simulink model "DevLib_PwrStgState"  (R2016b)
settings: configuration reference "CodeGenConfigSet" (kept outside this file)
values from neighbouring files (symbols this model uses):
  DebLib_facPwrStgHighHysHi_C = Calibration.Parameter    [init_DevLib_PwrStgState.m]
  DebLib_facPwrStgHighHysLo_C = Calibration.Parameter    [init_DevLib_PwrStgState.m]
  DebLib_facPwrStgLowHysHi_C = Calibration.Parameter    [init_DevLib_PwrStgState.m]
  DebLib_facPwrStgLowHysLo_C = Calibration.Parameter    [init_DevLib_PwrStgState.m]
  DebLib_uBattThdBattHiHysHi_C = Calibration.Parameter    [init_DevLib_PwrStgState.m]
  DebLib_uBattThdBattHiHysLo_C = Calibration.Parameter    [init_DevLib_PwrStgState.m]
  DebLib_uBattThdBattLoHysHi_C = Calibration.Parameter    [init_DevLib_PwrStgState.m]
  DebLib_uBattThdBattLoHysLo_C = Calibration.Parameter    [init_DevLib_PwrStgState.m]
  DebLib_uPwrStgBattHiHysHi_C = Calibration.Parameter    [init_DevLib_PwrStgState.m]
  DebLib_uPwrStgBattHiHysLo_C = Calibration.Parameter    [init_DevLib_PwrStgState.m]
  DebLib_uPwrStgBattLoHysHi_C = Calibration.Parameter    [init_DevLib_PwrStgState.m]
  DebLib_uPwrStgBattLoHysLo_C = Calibration.Parameter    [init_DevLib_PwrStgState.m]
undefined symbols (not defined in the file or in its folder): SubSysExeState_conv
libraries: simulink x13, CXLib x6
settings Model: Creator=lenovo  LastModifiedBy=lenovo
settings ConfigSetRef: SourceLocation=Base Workspace

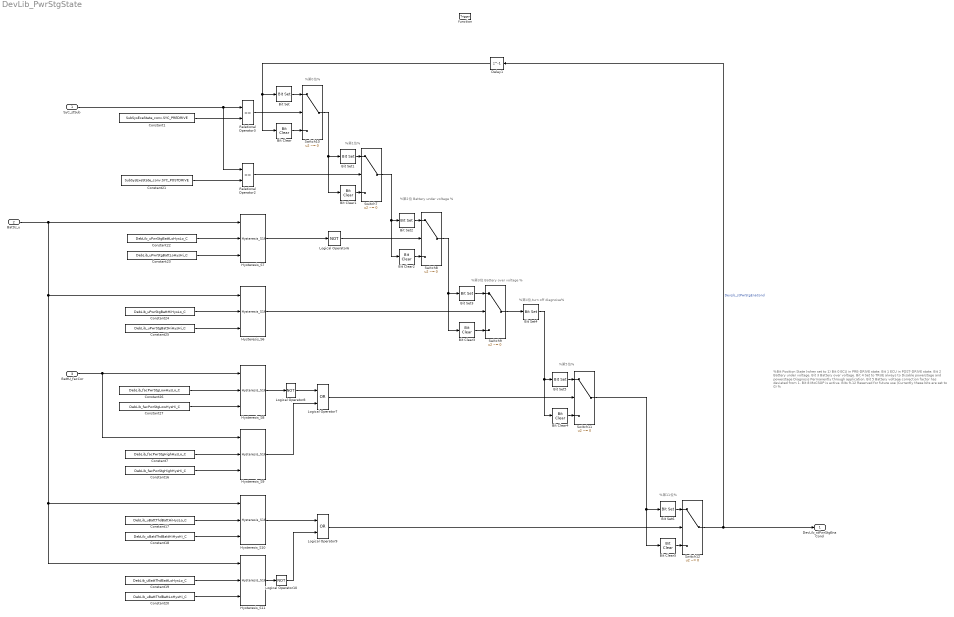
== system DevLib_PwrStgState ==
  note: %第11位%
  note: %第5位%
  note: %第4位,turn off diagnoise%
  note: %第3位 Battery over voltage %
  note: %第2位 Battery under voltage %
  note: %第1位%
  note: %第0位%
  note: %Bit Position State (when set to 1)
      | Bit 0 ECU in PRE-DRIVE state.
      | Bit 1 ECU in POST-DRIVE state.
      | Bit 2 Battery under voltage.
      | Bit 3 Battery over voltage.
      | Bit 4 Set to TRUE always to Disable powerstage and powerstage Diagnosis Permanently through application.
      | Bit 5 Battery voltage correction factor has deviated from 1.
      | Bit 8 MoCSOP is active.
      | Bits 9-12 Reserved for future use (Currently these bits are set to 0) %
  SyC_stSub : Inport  Description=Current system/ECU sub-state  OutDataTypeStr=Enum: SubSysExeState_conv
  BattU_u : Inport  Tag=mv  Description=Battery voltage  Port=2  OutMin=0  OutMax=50000  OutDataTypeStr=Battery_mv
  BattU_facCor : Inport  Description=Battery correction factor  Port=3  OutMin=-32  OutMax=31.9  OutDataTypeStr=Factor
  function : TriggerPort  TriggerType=function-call  VariantControl=Variant
  Bit Clear : simulink/Logic and Bit Operations/Bit Clear  iBit=0
  Bit Clear1 : simulink/Logic and Bit Operations/Bit Clear  iBit=1
  Bit Clear2 : simulink/Logic and Bit Operations/Bit Clear  iBit=2
  Bit Clear3 : simulink/Logic and Bit Operations/Bit Clear  iBit=3
  Bit Clear4 : simulink/Logic and Bit Operations/Bit Clear  iBit=5
  Bit Clear5 : simulink/Logic and Bit Operations/Bit Clear  iBit=11
  Bit Set : simulink/Logic and Bit Operations/Bit Set  iBit=0
  Bit Set1 : simulink/Logic and Bit Operations/Bit Set  iBit=1
  Bit Set2 : simulink/Logic and Bit Operations/Bit Set  iBit=2
  Bit Set3 : simulink/Logic and Bit Operations/Bit Set  iBit=3
  Bit Set4 : simulink/Logic and Bit Operations/Bit Set  iBit=4
  Bit Set5 : simulink/Logic and Bit Operations/Bit Set  iBit=5
  Bit Set6 : simulink/Logic and Bit Operations/Bit Set  iBit=11
  Constant1 : Constant  Value=SubSysExeState_conv.SYC_PREDRIVE  SampleTime=-1
  Constant16 : Constant  Value=DebLib_facPwrStgHighHysHi_C  SampleTime=-1
  Constant17 : Constant  Value=DebLib_uBattThdBattHiHysLo_C  VectorParams1D=off  SampleTime=-1
  Constant18 : Constant  Value=DebLib_uBattThdBattHiHysHi_C  SampleTime=-1
  Constant19 : Constant  Value=DebLib_uBattThdBattLoHysLo_C  VectorParams1D=off  SampleTime=-1
  Constant20 : Constant  Value=DebLib_uBattThdBattLoHysHi_C  SampleTime=-1
  Constant21 : Constant  Value=SubSysExeState_conv.SYC_POSTDRIVE  SampleTime=-1
  Constant22 : Constant  Value=DebLib_uPwrStgBattLoHysLo_C  SampleTime=-1
  Constant23 : Constant  Value=DebLib_uPwrStgBattLoHysHi_C  SampleTime=-1
  Constant24 : Constant  Value=DebLib_uPwrStgBattHiHysLo_C  SampleTime=-1
  Constant25 : Constant  Value=DebLib_uPwrStgBattHiHysHi_C  SampleTime=-1
  Constant26 : Constant  Value=DebLib_facPwrStgLowHysLo_C  SampleTime=-1
  Constant27 : Constant  Value=DebLib_facPwrStgLowHysHi_C  SampleTime=-1
  Constant7 : Constant  Value=DebLib_facPwrStgHighHysLo_C  SampleTime=-1
  Delay1 : Delay  DelayLength=1  InitialCondition=0
  Hysteresis_S{6..11} (6 alike) : CXLib/Hysteresis_S16
  Logical Operator10 : Logic  Operator=NOT  AllPortsSameDT=off  OutDataTypeStr=boolean
  Logical Operator6 : Logic  Operator=NOT  AllPortsSameDT=off  OutDataTypeStr=boolean
  Logical Operator7 : Logic  Operator=OR  AllPortsSameDT=off  OutDataTypeStr=boolean
  Logical Operator8 : Logic  Operator=NOT  AllPortsSameDT=off  OutDataTypeStr=boolean
  Logical Operator9 : Logic  Operator=OR  AllPortsSameDT=off  OutDataTypeStr=boolean
  Relational Operator2 : RelationalOperator  Operator===  OutDataTypeStr=boolean  RndMeth=Nearest  InputSameDT=on
  Relational Operator3 : RelationalOperator  Operator===  OutDataTypeStr=boolean  RndMeth=Nearest  InputSameDT=on
  Switch{7,9..12} (5 alike) : Switch  Criteria=u2 ~= 0  InputSameDT=on
  Switch8 : Switch  Criteria=u2 ~= 0
  DevLib_stPwrStgEnaCond : Outport  Description=Control unit status relevant to power stage deactivation/error diagnosis  OutMin=0  OutMax=65535  OutDataTypeStr=State_uint16
  wires:
  Constant1/1 -> Relational Operator3/2
  Constant21/1 -> Relational Operator2/2
  Constant22/1 -> Hysteresis_S7/2
  Constant23/1 -> Hysteresis_S7/3
  Constant24/1 -> Hysteresis_S6/2
  Constant25/1 -> Hysteresis_S6/3
  Constant26/1 -> Hysteresis_S8/2
  Constant27/1 -> Hysteresis_S8/3
  Constant7/1 -> Hysteresis_S9/2
  Constant16/1 -> Hysteresis_S9/3
  Constant20/1 -> Hysteresis_S11/3
  Constant19/1 -> Hysteresis_S11/2
  Constant18/1 -> Hysteresis_S10/3
  Constant17/1 -> Hysteresis_S10/2
  Logical Operator10/1 -> Logical Operator9/2
  Delay1/1 -> Bit Set/1, Bit Clear/1
  Bit Set6/1 -> Switch12/1
  Bit Clear5/1 -> Switch12/3
  Switch12/1 -> DevLib_stPwrStgEnaCond/1, Delay1/1  "DevLib_stPwrStgEnaCond"
  Logical Operator9/1 -> Switch12/2
  Switch11/1 -> Bit Set6/1, Bit Clear5/1
  Bit Clear4/1 -> Switch11/3
  Bit Set5/1 -> Switch11/1
  Bit Set4/1 -> Bit Set5/1, Bit Clear4/1
  Logical Operator7/1 -> Switch11/2
  Switch9/1 -> Bit Set4/1
  Bit Clear3/1 -> Switch9/3
  Bit Set3/1 -> Switch9/1
  Switch8/1 -> Bit Set3/1, Bit Clear3/1
  Hysteresis_S6/1 -> Switch9/2
  Bit Set2/1 -> Switch8/1
  Bit Clear2/1 -> Switch8/3
  Switch7/1 -> Bit Set2/1, Bit Clear2/1
  Logical Operator6/1 -> Switch8/2
  Switch10/1 -> Bit Set1/1, Bit Clear1/1
  Bit Clear1/1 -> Switch7/3
  Bit Set1/1 -> Switch7/1
  Relational Operator2/1 -> Switch7/2
  Bit Clear/1 -> Switch10/3
  Bit Set/1 -> Switch10/1
  Relational Operator3/1 -> Switch10/2
  Hysteresis_S11/1 -> Logical Operator10/1
  Hysteresis_S10/1 -> Logical Operator9/1
  Hysteresis_S9/1 -> Logical Operator7/2
  Hysteresis_S8/1 -> Logical Operator8/1
  BattU_facCor/1 -> Hysteresis_S9/1, Hysteresis_S8/1
  Logical Operator8/1 -> Logical Operator7/1
  Hysteresis_S7/1 -> Logical Operator6/1
  BattU_u/1 -> Hysteresis_S7/1, Hysteresis_S6/1, Hysteresis_S10/1, Hysteresis_S11/1
  SyC_stSub/1 -> Relational Operator3/1, Relational Operator2/1
